simulink model "Expriment_All3"  (R2014a)
settings: Solver=FixedStepDiscrete  SolverMode=SingleTasking  StartTime=0.0  StopTime=inf  FixedStep=0.01  RelTol=1e-3
PostLoadFcn:
  | h_RPStest = RPStest;
model workspace (MAT data in the model file):
  gtest = 0
undefined symbols (not defined in the file or in its folder): avert, avert_freq_factor, avert_gaze_dirs_chance, avert_gaze_duration_factor, avert_head_frequency_factor, avert_head_speed, BML, BML1, BML2, bmlsL, bmlsM, bodyBusyFlag, clock, emotion_amount_factor, faceBusyFlag, fileID, GAZE_WIN, gazing, head_mut_chance, mut_freq_factor, mutual_gaze_duration_factor, P, pose_cat_chance, pose_chanc_factor, pose_chance_factor, pose_frequency_factor, pose_lean, pose_lean_flag, pose_speed, pose_twitch, pr, serial, STATE_BEFORE, STATE_GO, STATE_OVER, STATE_READY, Stateflow
libraries: simulink x24, instrumentlib x6, lib_affectiveChar_behavior x3, realtime_pacer_lib x2, lib_affectiveChar_input x1
(part 7 of 7)

== matlab function Expriment_All3/EmotionSubsystem/calculateValenceArousal/LEHN_A ==
  data: a2 output double size=1; a1 input double size=1
function a2 = fcn(a1)

aVarTruthTableCondition_1 = false;
aVarTruthTableCondition_2 = false;



aVarTruthTableCondition_1 = logical(a1>25);


aVarTruthTableCondition_2 = logical(a1<-25);

if (aVarTruthTableCondition_1)
    aFcnTruthTableAction_1();
elseif (aVarTruthTableCondition_2)
    aFcnTruthTableAction_2();
else % Default
    aFcnTruthTableAction_3();
end

function aFcnTruthTableAction_1()


a2=a1;

function aFcnTruthTableAction_2()


a2=a1;

function aFcnTruthTableAction_3()


a2=0;

== stateflow chart Expriment_All3/CharacterControl/custom_Behavior_Factors ==
  state setP
    entry:
    [mutual_gaze_duration_factor, avert_gaze_duration_factor,avert_head_frequency_factor,avert_head_speed,avert_gaze_dirs_chance,avert_freq_factor,mut_freq_factor,head_mut_chance]=sharedFunc.setGazeFactors(inV,inA,personality,personalityFlag,vaFlag,gazeArray,personalityChange);
  state init
    entry: mutual_gaze_duration_factor=1;avert_gaze_duration_factor=1;head_mut_chance=60;
    avert_head_frequency_factor=30;avert_head_speed=1;avert_gaze_dirs_chance=1;,avert_freq_factor=1;mut_freq_factor=1;
    pose_frequency_factor=30;pose_chanc_factor=1;pose_cat_chance=10;pose_lean=10;pose_speed=1;pose_lean_flag=0;
  state wait
  state sharedFunc [group]
  state setP1
    entry:
    [pose_twitch,pose_frequency_factor,pose_chanc_factor,pose_cat_chance,pose_lean,pose_speed,pose_lean_flag]=sharedFunc.setPoseFactors(inV,inA,personality,personalityFlag,vaFlag,poseArray,personalityChange);
  (default) -> init
  init -> wait
  wait -> setP [order 1] : [gazeArray(:,1)==1]
  setP -> wait
  setP1 -> wait
  wait -> setP1 [order 2] : [poseArray(:,1)==1]
  data: inA input double size=1; inV input double size=1; vaFlag input boolean size=1; personalityFlag input boolean size=1; gazeArray input double size=[1, 6]; personality input double size=1; personalityChange input boolean size=1; mutual_gaze_duration_factor data_store_memory; avert_head_frequency_factor data_store_memory; avert_gaze_duration_factor data_store_memory; avert_head_speed data_store_memory; avert_gaze_dirs_chance data_store_memory; poseArray input double size=[1, 6]; pose_lean data_store_memory; pose_speed data_store_memory; pose_chanc_factor data_store_memory; pose_frequency_factor data_store_memory; pose_cat_chance data_store_memory; pose_lean_flag data_store_memory; emotion_amount_custom input double size=1; emotion_amount_factor data_store_memory size=1; mut_freq_factor data_store_memory; avert_freq_factor data_store_memory; pose_twitch data_store_memory; head_mut_chance data_store_memory

== matlab function Expriment_All3/EmotionSubsystem/calculateValenceArousal/LEHN plot ==
  data: v input; a input
function fcn(v,a)
%coder.extrinsic to bypass code generation
coder.extrinsic('fscanf')
coder.extrinsic('get_param');
% coder.extrinsic('importdata');

currentTime=get_param('Expriment_FacialExpr','SimulationTime');%use name of simulink proj

A = [v;a;currentTime];

fileID = fopen('LEHN_VA_table.txt','a');
fprintf(fileID,'%0.1f,%0.1f,%0.1f\r\n',A);
fclose(fileID);

%use the following to draw the plot
%tmp_data = importdata('HEHN_VA_table.txt',','); 
%no need: x=tmp_data(:,1);y=tmp_data(:,2);z=tmp_data(:,3)
%matrix=tmp_data
%tri = delaunay(matrix(:,1),matrix(:,2));
%trisurf(tri,matrix(:,1),matrix(:,2),matrix(:,3))
%shading interp

%-----------------------------------------
% fileID = fopen('HEHN_VA_table.txt','r');
% formatSpec = '%1f\r %1f\r %1f\r\n';
% sizeA = [3 Inf];
% A = fscanf(fileID,formatSpec,sizeA)
% % A = A'
% fclose(fileID);

% x = zeros(100,2);y = zeros(100,2);
% filename = 'HEHN_VA_table.txt';
% delimiterIn = ' ';
% headerlinesIn = 1;
% A = importdata(filename,delimiterIn,headerlinesIn);

% fileID=fopen('HEHN_VA_table4.txt');
% s=textscan(fileID,'%d %d %d','headerlines',23);
% fclose(fileID);
% x=s{1}

== matlab function Expriment_All3/EmotionSubsystem/calculateValenceArousal/LELN plot ==
  data: v input; a input
function fcn(v,a)
%coder.extrinsic to bypass code generation
coder.extrinsic('fscanf')
coder.extrinsic('get_param');
% coder.extrinsic('importdata');

currentTime=get_param('Expriment_FacialExpr','SimulationTime');%use name of simulink proj

A = [v;a;currentTime];

fileID = fopen('LELN_VA_table.txt','a');
fprintf(fileID,'%0.1f,%0.1f,%0.1f\r\n',A);
fclose(fileID);

%use the following to draw the plot
%matrix = importdata('HEHN_VA_table.txt',','); 
%tri = delaunay(matrix(:,1),matrix(:,2));
%trisurf(tri,matrix(:,1),matrix(:,2),matrix(:,3))
%shading interp
%colorbar
%-----------------------------------------
% fileID = fopen('HEHN_VA_table.txt','r');
% formatSpec = '%1f\r %1f\r %1f\r\n';
% sizeA = [3 Inf];
% A = fscanf(fileID,formatSpec,sizeA)
% % A = A'
% fclose(fileID);

% x = zeros(100,2);y = zeros(100,2);
% filename = 'HEHN_VA_table.txt';
% delimiterIn = ' ';
% headerlinesIn = 1;
% A = importdata(filename,delimiterIn,headerlinesIn);

% fileID=fopen('HEHN_VA_table4.txt');
% s=textscan(fileID,'%d %d %d','headerlines',23);
% fclose(fileID);
% x=s{1}

== matlab function Expriment_All3/EmotionSubsystem/calculateValenceArousal/LEHN_V ==
  data: v2 output double size=1; v1 input double size=1
function v2 = fcn(v1)

aVarTruthTableCondition_1 = false;
aVarTruthTableCondition_2 = false;



aVarTruthTableCondition_1 = logical(v1>25);


aVarTruthTableCondition_2 = logical(v1<-25);

if (aVarTruthTableCondition_1)
    aFcnTruthTableAction_1();
elseif (aVarTruthTableCondition_2)
    aFcnTruthTableAction_2();
else % Default
    aFcnTruthTableAction_3();
end

function aFcnTruthTableAction_1()


v2=v1;

function aFcnTruthTableAction_2()


v2=v1;

function aFcnTruthTableAction_3()


v2=0;

== matlab function Expriment_All3/EmotionSubsystem/calculateValenceArousal/LELN_A ==
  data: a2 output double size=1; a1 input double size=1
function a2 = fcn(a1)

aVarTruthTableCondition_1 = false;
aVarTruthTableCondition_2 = false;



aVarTruthTableCondition_1 = logical(a1>25);


aVarTruthTableCondition_2 = logical(a1<-25);

if (aVarTruthTableCondition_1)
    aFcnTruthTableAction_1();
elseif (aVarTruthTableCondition_2)
    aFcnTruthTableAction_2();
else % Default
    aFcnTruthTableAction_3();
end

function aFcnTruthTableAction_1()


a2=a1;

function aFcnTruthTableAction_2()


a2=a1;

function aFcnTruthTableAction_3()


a2=0;

== matlab function Expriment_All3/EmotionSubsystem/calculateValenceArousal/LELN_VA_Emo ==
  data: V input; e output double size=1; A input double
function e = fcn(V, A)

aVarTruthTableCondition_1 = false;
aVarTruthTableCondition_2 = false;
aVarTruthTableCondition_3 = false;
aVarTruthTableCondition_4 = false;
aVarTruthTableCondition_5 = false;
aVarTruthTableCondition_6 = false;
aVarTruthTableCondition_7 = false;
aVarTruthTableCondition_8 = false;


% 7-happy  2,1

aVarTruthTableCondition_1 = logical(V>20 && A<40 && A>20);

% 8-ex  1,2 AND 2,2

aVarTruthTableCondition_2 = logical(V>0 && A>40);

% 4-fear  -1,2 AND -2,2

aVarTruthTableCondition_3 = logical(V<0 && A>40);

% 3-frust  -2,1

aVarTruthTableCondition_4 = logical(V<-20 && A<40 && A>20);

% 6-idle  2,-1

aVarTruthTableCondition_5 = logical(V>20 && A<-20 && A>-40);

% 5-calm  1,-2 AND 2,-2

aVarTruthTableCondition_6 = logical(V>0 && A<-40);

% 1-bored  -1,-2 AND -2,-2

aVarTruthTableCondition_7 = logical(V<0 && A<-40);

% 2-sad  -2,-1

aVarTruthTableCondition_8 = logical(V<-20 && A<-20 && A>-40);

if (aVarTruthTableCondition_1)
    aFcnTruthTableAction_1();
elseif (aVarTruthTableCondition_2)
    aFcnTruthTableAction_2();
elseif (aVarTruthTableCondition_3)
    aFcnTruthTableAction_3();
elseif (aVarTruthTableCondition_4)
    aFcnTruthTableAction_4();
elseif (aVarTruthTableCondition_5)
    aFcnTruthTableAction_5();
elseif (aVarTruthTableCondition_6)
    aFcnTruthTableAction_6();
elseif (aVarTruthTableCondition_7)
    aFcnTruthTableAction_7();
elseif (aVarTruthTableCondition_8)
    aFcnTruthTableAction_8();
else % Default
    aFcnTruthTableAction_5();
end

function aFcnTruthTableAction_1()

% happy

e=7;

function aFcnTruthTableAction_2()

% excited

e=8;

function aFcnTruthTableAction_3()

% fear

e=4;

function aFcnTruthTableAction_4()

% frustration

e=3;

function aFcnTruthTableAction_5()

% idle

e=6;

function aFcnTruthTableAction_6()

% contempt

e=5;

function aFcnTruthTableAction_7()

% bored

e=1;

function aFcnTruthTableAction_8()

% sad

e=2;

== matlab function Expriment_All3/EmotionSubsystem/satFunction ==
  data: randv input; smile input; wave input; win input; invade input; v_trigW output; vaFlag input; v_trig output
function [v_trigW,v_trig]= fcn(randv,smile,wave,win,invade,vaFlag)
%#codegen
% 30/06/2015
    %Here set Agent's satisfaction flag based on your scenario
    %In RPS scenario agent gets satisfined when she wins. states of interaction= {STATE_READY=7;
    %STATE_GO=1;STATE_HAND=2;STATE_OVER=3; STATE_BEFORE=4;STATE_RESULT=5;STATE_WAIT=6;}
   
    if(vaFlag==1)
        v_trigW=0;%weight by which valence value is changed (sum of weight of all triggers)
        %randv 30% chance of random increase or decrease in valence
        randTrigger=floor(randv);
        if(0<randTrigger)&&(randTrigger<30)
            v_trigW = v_trigW + 0.6;
        end
        if(30<randTrigger)&&(randTrigger<60)
            v_trigW = v_trigW - 0.6;
        end

        if(win==2) %agent wins so she is satisfied
            v_trigW = v_trigW + 0.5;
        elseif(win==1) %user wins so agent is NOT satisfied
            v_trigW = v_trigW - 0.5;
        end

        if(smile==1)
            v_trigW=v_trigW+0.25;
        end

        if(wave==1)
            v_trigW=v_trigW+0.25;
        end

        if(invade==1)
            v_trigW=v_trigW-0.25;
        end
    else
         v_trigW=0;
    end
    if(v_trigW>0)
        v_trig=1;
    elseif(v_trigW<0)
        v_trig=-1;
        v_trigW=abs(v_trigW);
    else
        v_trig=0;
    end
